simulink model "RpiScopeRun"  (R2023a)
settings: Solver=VariableStepAuto  StartTime=0.0  StopTime=48  RelTol=1e-3
libraries: embmathops x2, simulink x1
settings Model: Creator=umphaipunatipunumphai  LastModifiedBy=umphaipunatipunumphai

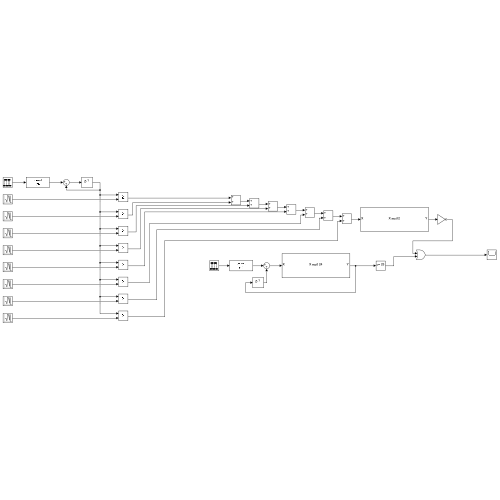
[thumbnail: Simulink's stored preview of the top-level diagram]
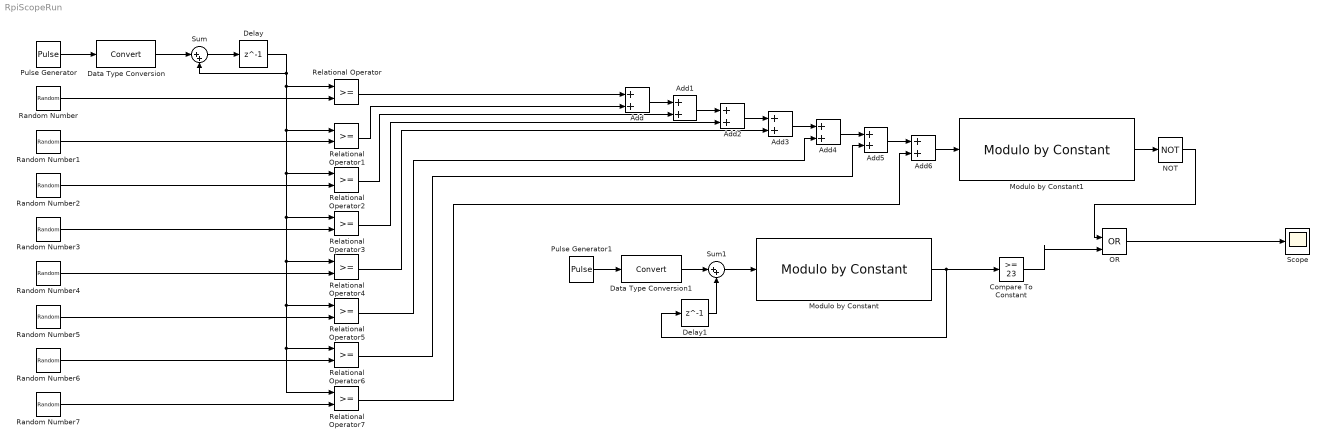
== system RpiScopeRun ==
  Add{,1..6} (7 alike) : Sum
  Compare To Constant : simulink/Logic and Bit Operations/Compare To Constant  relop=>=  const=23  OutDataTypeStr=boolean
  Data Type Conversion : DataTypeConversion  OutMin=0  OutMax=1  ConvertRealWorld=Stored Integer (SI)  RndMeth=Nearest  SaturateOnIntegerOverflow=off
  Data Type Conversion1 : DataTypeConversion  OutMin=0  OutMax=1  ConvertRealWorld=Stored Integer (SI)  RndMeth=Nearest  SaturateOnIntegerOverflow=off
  Delay : Delay  DelayLength=1  InitialCondition=0  SampleTime=1
  Delay1 : Delay  DelayLength=1  InitialCondition=0  SampleTime=1
  Modulo by Constant : embmathops/Modulo by Constant  Denominator=24  SimulateUsing=Code generation
      settings: LibrarySourceBlock=embeddedMathLib/Modulo by Constant
  Modulo by Constant1 : embmathops/Modulo by Constant  Denominator=2  SimulateUsing=Code generation
      settings: LibrarySourceBlock=embeddedMathLib/Modulo by Constant
  NOT : Logic  Operator=NOT  IconShape=distinctive  AllPortsSameDT=off  OutDataTypeStr=boolean
  OR : Logic  Operator=OR  IconShape=distinctive  AllPortsSameDT=off  OutDataTypeStr=boolean
  Pulse Generator : DiscretePulseGenerator  Period=1  SampleTime=48
  Pulse Generator1 : DiscretePulseGenerator  Period=1  SampleTime=48
  Random Number : RandomNumber  Mean=3  SampleTime=48
  Random Number1 : RandomNumber  Mean=9  Seed=1  SampleTime=48
  Random Number2 : RandomNumber  Mean=15  Seed=2  SampleTime=48
  Random Number3 : RandomNumber  Mean=21  Seed=3  SampleTime=48
  Random Number4 : RandomNumber  Mean=27  Seed=4  SampleTime=48
  Random Number5 : RandomNumber  Mean=33  Seed=5  SampleTime=48
  Random Number6 : RandomNumber  Mean=39  Seed=6  SampleTime=48
  Random Number7 : RandomNumber  Mean=45  Seed=7  SampleTime=48
  Relational Operator{,1..7} (8 alike) : RelationalOperator  OutDataTypeStr=boolean  RndMeth=Simplest  InputSameDT=off
  Scope : Scope
  Sum : Sum  Inputs=|++
  Sum1 : Sum  Inputs=|++
  wires:
  Random Number3/1 -> Relational Operator3/2
  Random Number7/1 -> Relational Operator7/2
  Random Number1/1 -> Relational Operator1/2
  Random Number5/1 -> Relational Operator5/2
  Random Number6/1 -> Relational Operator6/2
  Random Number/1 -> Relational Operator/2
  Random Number2/1 -> Relational Operator2/2
  Random Number4/1 -> Relational Operator4/2
  Pulse Generator/1 -> Data Type Conversion/1
  Data Type Conversion/1 -> Sum/1
  Delay/1 -> Relational Operator/1, Relational Operator6/1, Relational Operator7/1, Relational Operator5/1, Relational Operator4/1, Relational Operator3/1, Relational Operator2/1, Relational Operator1/1, Sum/2
  Sum/1 -> Delay/1
  Compare To Constant/1 -> OR/2
  Relational Operator/1 -> Add/1
  Relational Operator4/1 -> Add3/2
  Modulo by Constant/1 -> Compare To Constant/1, Delay1/1
  Add4/1 -> Add5/1
  Relational Operator6/1 -> Add5/2
  Add3/1 -> Add4/1
  Relational Operator5/1 -> Add4/2
  Add1/1 -> Add2/1
  Add5/1 -> Add6/1
  Relational Operator1/1 -> Add/2
  Delay1/1 -> Sum1/2
  Relational Operator2/1 -> Add1/2
  Add/1 -> Add1/1
  Add2/1 -> Add3/1
  Relational Operator7/1 -> Add6/2
  Add6/1 -> Modulo by Constant1/1
  Data Type Conversion1/1 -> Sum1/1
  Relational Operator3/1 -> Add2/2
  Modulo by Constant1/1 -> NOT/1
  NOT/1 -> OR/1
  Sum1/1 -> Modulo by Constant/1
  Pulse Generator1/1 -> Data Type Conversion1/1
  OR/1 -> Scope/1
